simulink model "delta_w_minus"  (Simulink 7.8)
settings: Solver=ode45  StartTime=0.0  StopTime=10.0  RelTol=1e-3
settings Model: Creator=Leo  LastModifiedBy=Leo

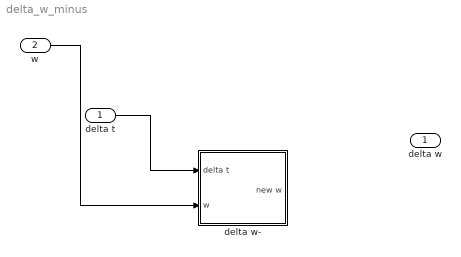
== system delta_w_minus ==
  delta t : Inport
  w : Inport  Port=2
  delta w- : Subsystem
  delta w : Outport
  wires:
  delta t/1 -> delta w-/1(delta t)
  w/1 -> delta w-/2(w)
  ? -> delta w/1

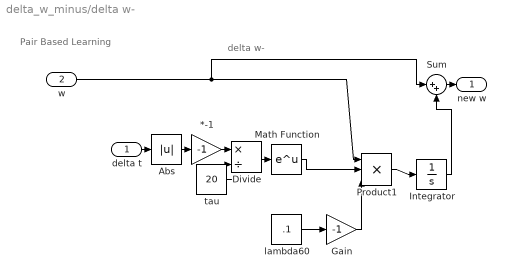
== system delta_w_minus/delta w- ==
  note: Pair Based Learning
  note: delta w-
  delta t : Inport
  w : Inport  Port=2
  *-1 : Gain  Gain=-1
  Abs : Abs
  Divide : Product  Inputs=*/
  Gain : Gain  Gain=-1
  Integrator : Integrator
  Math Function : Math  SaturateOnIntegerOverflow=on
  Product1 : Product  Inputs=***
  Sum : Sum  Inputs=|++
  lambda60 : Constant  Value=.1
  tau : Constant  Value=20
  new w : Outport
  wires:
  delta t/1 -> Abs/1
  Abs/1 -> *-1/1
  *-1/1 -> Divide/1
  tau/1 -> Divide/2
  Divide/1 -> Math Function/1
  w/1 -> Product1/1, Sum/1
  lambda60/1 -> Gain/1
  Math Function/1 -> Product1/2
  Gain/1 -> Product1/3
  Product1/1 -> Integrator/1
  Integrator/1 -> Sum/2
  Sum/1 -> new w/1
